simulink model "Saturation"  (R2023b)
settings: Solver=VariableStepAuto  StartTime=0.0  StopTime=10.0  RelTol=1e-3
settings Model: Creator=hp  LastModifiedBy=hp

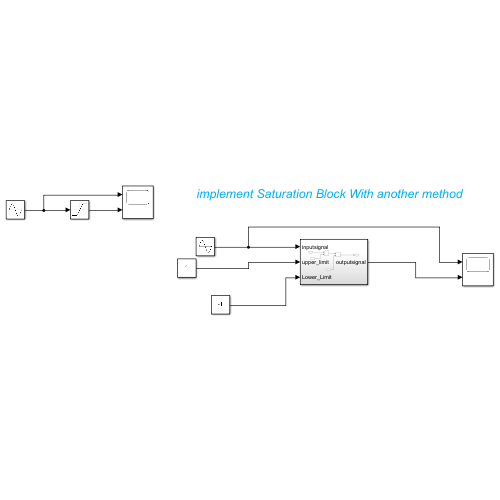
[thumbnail: Simulink's stored preview of the top-level diagram]
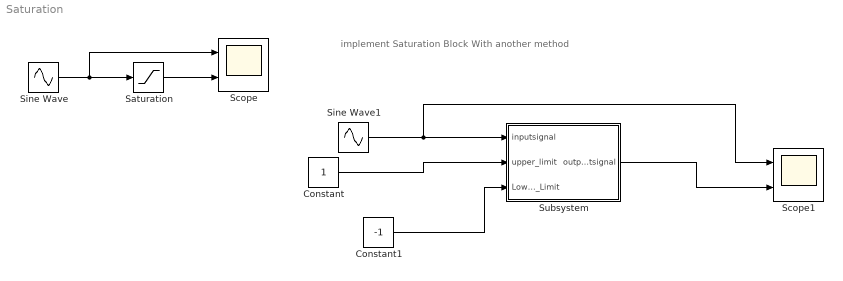
== system Saturation ==
  note: implement Saturation Block With another method
  Constant : Constant
  Constant1 : Constant  Value=-1
  Saturation : Saturate  UpperLimit=1  LowerLimit=-1
  Scope : Scope  NumInputPorts=2
  Scope1 : Scope  NumInputPorts=2
  Sine Wave : Sin  Amplitude=2  SampleTime=0
  Sine Wave1 : Sin  Amplitude=2  SampleTime=0
  Subsystem : Subsystem
  wires:
  Sine Wave/1 -> Scope/1, Saturation/1
  Saturation/1 -> Scope/2
  Sine Wave1/1 -> Subsystem/1(inputsignal), Scope1/1
  Constant/1 -> Subsystem/2(upper_limit)
  Constant1/1 -> Subsystem/3(Lower_Limit)
  Subsystem/1(outputsignal) -> Scope1/2

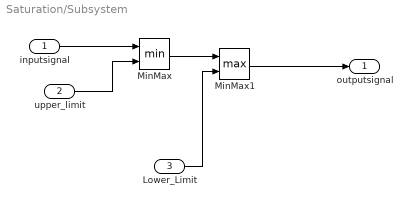
== system Saturation/Subsystem ==
  inputsignal : Inport
  upper_limit : Inport  Port=2
  Lower_Limit : Inport  Port=3
  MinMax : MinMax  Inputs=2
  MinMax1 : MinMax  Function=max  Inputs=2
  outputsignal : Outport
  wires:
  MinMax/1 -> MinMax1/1
  MinMax1/1 -> outputsignal/1
  inputsignal/1 -> MinMax/1
  Lower_Limit/1 -> MinMax1/2
  upper_limit/1 -> MinMax/2
